simulink model "foc"  (R2021b)
settings: Solver=FixedStepAuto  StartTime=0.0  StopTime=20  FixedStep=Ts  MaxStep=1e-4  RelTol=1e-3
values from neighbouring files (symbols this model uses):
  currt_width = 200.0    [motor_parameters.sldd]
  Flux = 0.00103001    [motor_parameters.sldd]
  Gamma = 800000.0    [motor_parameters.sldd]
  Ibus = 5.0    [motor_parameters.sldd]
  Ls = 2.235E-5    [motor_parameters.sldd]
  Pn = 7.0    [motor_parameters.sldd]
  Rs = 0.112    [motor_parameters.sldd]
  Ts = 0.0001    [motor_parameters.sldd]
  Ubus = 12.0    [motor_parameters.sldd]
undefined symbols (not defined in the file or in its folder): DiscIntNeverNeededParam, magnitude, sigbuilder_block, spd_ki, spd_kp
libraries: slpidlib x4, mcbplantlib x1, simulink x1, autolibpmsmexterior x1
settings Model: DataDictionary=motor_parameters.sldd  Creator=chenpeng  LastModifiedBy=chenpeng
settings SolverCC: AutoInsertRateTranBlk=on
settings OptimizationCC: DefaultParameterBehavior=Inlined  UseDivisionForNetSlopeComputation=on  GainParamInheritBuiltInType=on  UseFloatMulNetSlope=on  InlineInvariantSignals=on  PassReuseOutputArgsAs=Individual arguments  ZeroExternalMemoryAtStartup=off  ZeroInternalMemoryAtStartup=off  NoFixptDivByZeroProtection=on  EfficientFloat2IntCast=on  LifeSpan=1  OptimizeBlockOrder=speed  DifferentSizesBufferReuse=on  EfficientTunableParamExpr=on
settings DebuggingCC: ParameterTunabilityLossMsg=error
settings HardwareCC: ProdBitPerPointer=32  ProdBitPerSizeT=32  ProdBitPerPtrDiffT=32  ProdLargestAtomicInteger=Long  ProdLargestAtomicFloat=Double  ProdWordSize=32  ProdLongLongMode=on  ProdHWDeviceType=ARM Compatible->ARM Cortex-M
settings SFSimCC: MATLABDynamicMemAlloc=off
settings RTWCC: Description=Embedded Coder  SystemTargetFile=ert.tlc  GenCodeOnly=on  TemplateMakefile=ert_default_tmf  Toolchain=GNU Tools for ARM Embedded Processors
settings CodeAppCC: ForceParamTrailComments=on  IgnoreCustomStorageClasses=off  OperatorAnnotations=on  SimulinkDataObjDesc=on  SFDataObjDesc=on  CustomSymbolStrGlobalVar=rt$N$M  CustomSymbolStrType=$N$M  CustomSymbolStrFcn=$N$M$F  CustomSymbolStrMacro=$N$M  InsertBlockDesc=on
settings ERTTargetCC: TargetLangStandard=C99 (ISO)  GenerateSampleERTMain=on  IncludeMdlTerminateFcn=off  CombineSignalStateStructs=on  SupportComplex=off  SupportNonInlinedSFcns=on  InlinedParameterPlacement=NonHierarchical  ERTCustomFileTemplate=example_file_process.tlc  ERTFilePackagingFormat=CompactWithDataFile

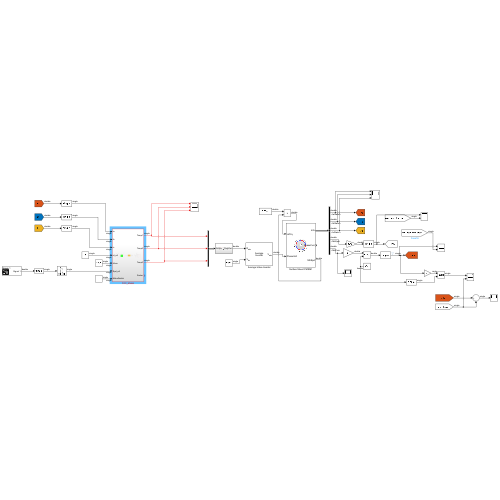
[thumbnail: Simulink's stored preview of the top-level diagram]
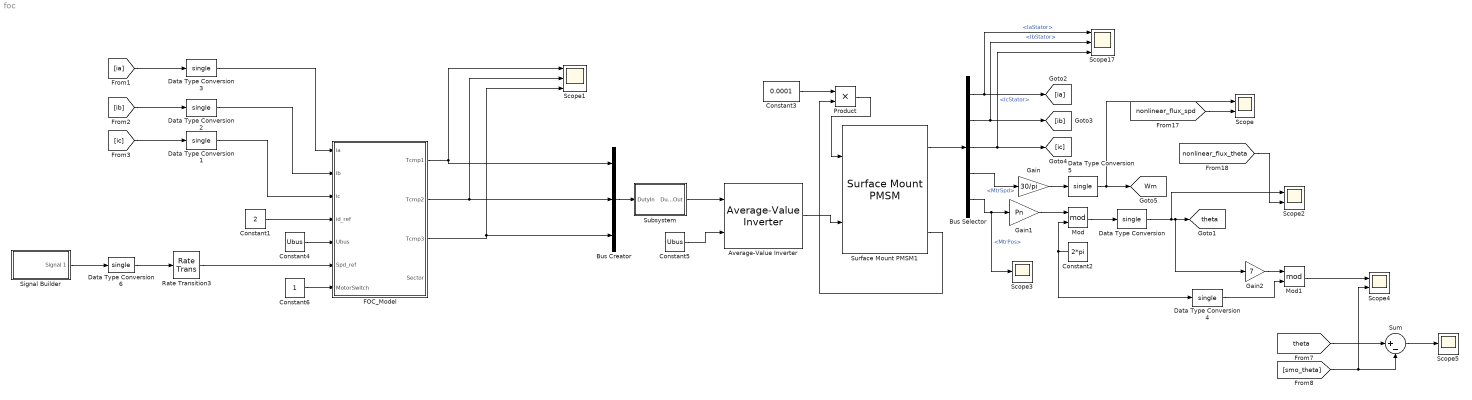
== system foc ==
  Average-Value Inverter : mcbplantlib/Average-Value Inverter
  Bus Creator : BusCreator  Inputs=3
  Bus Selector : BusSelector  OutputSignals=IaStator,IbStator,IcStator,MtrSpd,MtrPos
  Constant1 : Constant  Value=2  OutDataTypeStr=single  SampleTime=-1
  Constant2 : Constant  Value=2*pi
  Constant3 : Constant  Value=0.0001  OutDataTypeStr=double
  Constant4 : Constant  Value=Ubus  OutDataTypeStr=single
  Constant5 : Constant  Value=Ubus  OutDataTypeStr=single
  Constant6 : Constant  OutDataTypeStr=single  SampleTime=-1
  Data Type Conversion{,1..6} (7 alike) : DataTypeConversion  OutDataTypeStr=single
  FOC_Model : Subsystem
  Gain : Gain  Gain=30/pi
  Gain1 : Gain  Gain=Pn
  Gain2 : Gain  Gain=7
  Mod : Math  Operator=mod  SaturateOnIntegerOverflow=on
  Mod1 : Math  Operator=mod  SaturateOnIntegerOverflow=on
  Product : Product
  Rate Transition3 : RateTransition
  Scope : Scope  NumInputPorts=2
  Scope1 : Scope  NumInputPorts=3
  Scope17 : Scope  NumInputPorts=3
  Scope2 : Scope  NumInputPorts=2
  Scope3 : Scope
  Scope4 : Scope  NumInputPorts=2
  Scope5 : Scope
  Signal Builder : Subsystem  Tag=STV Subsys  LoadFcn=sigbuilder_block('load');  StartFcn=sigbuilder_block('start');  StopFcn=sigbuilder_block('stop');  ClipboardFcn=sigbuilder_block('clipboard');  mask(Sigbuilder block){tuvar=[0:10]}
      mask help: Simulink:masks:SigbuilderBlock_MD
      mask init:
      | if ~strcmp(get_param(bdroot(gcbh),'SimulationStatus'),'stopped') tuvar = sigbuilder_block('maskInit'); end
      settings: CopyFcn=sigbuilder_block('copy');  DeleteFcn=sigbuilder_block('delete');  ModelCloseFcn=sigbuilder_block('modelClose');  PreSaveFcn=sigbuilder_block('preSave');  PauseFcn=sigbuilder_block('pause');  ContinueFcn=sigbuilder_block('continue');  NameChangeFcn=sigbuilder_block('namechange');  OpenFcn=sigbuilder_block('open',[437.6 199.2 550.4 400 ]);  CloseFcn=sigbuilder_block('close');
      mask Display: plot(0, 0, 100, 100,[2, 2, 32, 32, 2], [68, 8, 8, 68, 68],[32, 2], [38, 38], [32, 19, 2],[53, 60, 44], [32, 17, 17, 2],[16, 16, 31, 31]);txt = getActiveGroup(gcbh);text(2, 100, txt,'verticalAlignment', 'top');
  Subsystem : Subsystem
  Sum : Sum  Inputs=|+-
  Surface Mount PMSM1 : autolibpmsmexterior/Surface Mount PMSM  port_config=Torque  sim_type=Discrete  Ts=Ts  FilePath=E:\Sandbox\Bauto\Work\surfacepmsm_motordata.m  P=Pn  Rs=Rs  Ldq_=Ls  KConstText=Permanent flux linkage constant (lambda_pm):  lambda_pm=Flux  Ke=159.9771  Kt=1.323  mechanical=[0.0027, 4.924e-4, 0]  idq0=[0 0]  theta_init=0  omega_init=0  KConst=Flux  lambda_pm_calc=Flux  RefBlkName='autolibpmsmexterior/Surface Mount PMSM'  aMode=1  Ldq="[0.0003752   0.0003752]"
      settings: SourceProductBaseCode=PW,DR,MT,UV,VE
  tag scope: Wm=global, theta=global
  wires:
  Data Type Conversion/1 -> Scope2/1, Gain2/1, [theta]
  Bus Selector/3 -> Scope17/3, [ic]  "<IcStator>"
  Mod/1 -> Data Type Conversion/1
  Gain/1 -> Data Type Conversion5/1
  Constant3/1 -> Product/1
  Gain1/1 -> Mod/1
  Data Type Conversion5/1 -> Scope/1, [Wm]
  Bus Creator/1 -> Subsystem/1(DutyIn)
  Bus Selector/5 -> Scope3/1, Gain1/1  "<MtrPos>"
  Bus Selector/1 -> [ia], Scope17/1  "<IaStator>"
  Subsystem/1(DutyOut) -> Average-Value Inverter/1
  Bus Selector/2 -> Scope17/2, [ib]  "<IbStator>"
  Bus Selector/4 -> Gain/1  "<MtrSpd>"
  Constant2/1 -> Data Type Conversion4/1, Mod/2
  Constant5/1 -> Average-Value Inverter/2
  [ia] -> Data Type Conversion3/1
  [ib] -> Data Type Conversion2/1
  [ic] -> Data Type Conversion1/1
  Average-Value Inverter/1 -> Surface Mount PMSM1/2
  Surface Mount PMSM1/3 -> Product/2
  Surface Mount PMSM1/1 -> Bus Selector/1
  Gain2/1 -> Mod1/1
  Mod1/1 -> Scope4/1
  Data Type Conversion4/1 -> Mod1/2
  Product/1 -> Surface Mount PMSM1/1
  Data Type Conversion3/1 -> FOC_Model/1(ia)
  Data Type Conversion2/1 -> FOC_Model/2(ib)
  Data Type Conversion1/1 -> FOC_Model/3(ic)
  Constant4/1 -> FOC_Model/5(Ubus)
  FOC_Model/1(Tcmp1) -> Bus Creator/1, Scope1/1
  FOC_Model/2(Tcmp2) -> Scope1/2, Bus Creator/2
  FOC_Model/3(Tcmp3) -> Scope1/3, Bus Creator/3
  Constant6/1 -> FOC_Model/7(MotorSwitch)
  Constant1/1 -> FOC_Model/4(id_ref)
  [smo_theta] -> Scope4/2, Sum/2
  Sum/1 -> Scope5/1
  Data Type Conversion6/1 -> Rate Transition3/1
  Signal Builder/1(Signal 1) -> Data Type Conversion6/1
  [theta] -> Sum/1
  [nonlinear_flux_spd] -> Scope/2
  [nonlinear_flux_theta] -> Scope2/2
  Rate Transition3/1 -> FOC_Model/6(Spd_ref)

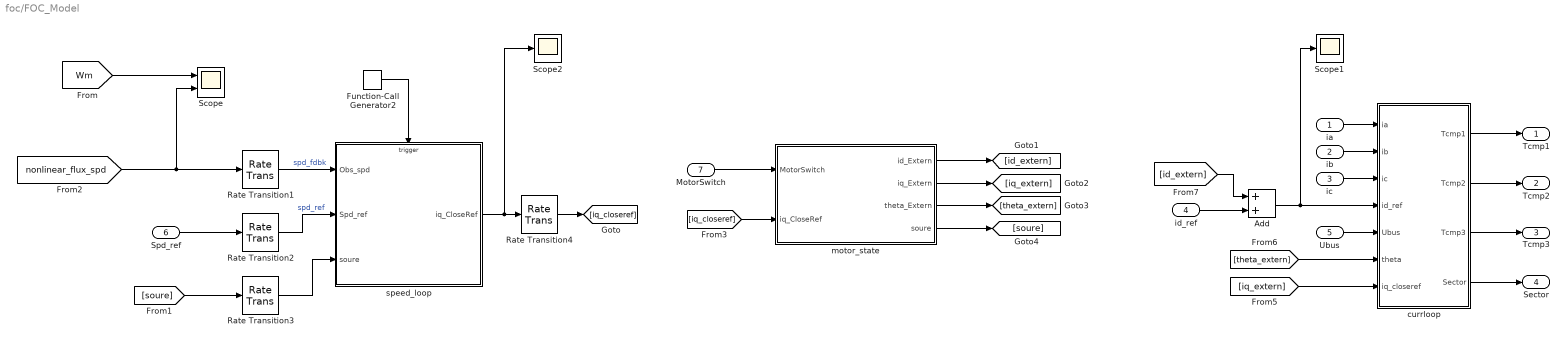
== system foc/FOC_Model ==
  ia : Inport  OutDataTypeStr=single
  ib : Inport  Port=2  OutDataTypeStr=single
  ic : Inport  Port=3  OutDataTypeStr=single
  id_ref : Inport  Port=4  OutDataTypeStr=single
  Ubus : Inport  Port=5  OutDataTypeStr=single
  Spd_ref : Inport  Port=6  OutDataTypeStr=single
  MotorSwitch : Inport  Port=7  OutDataTypeStr=single
  Add : Sum
  Function-Call Generator2 : simulink/Ports & Subsystems/Function-Call Generator  sample_time=1e-3  numberOfIterations=1  DisallowWideOutput=off
  Rate Transition{1..4} (4 alike) : RateTransition
  Scope : Scope  NumInputPorts=2
  Scope1 : Scope
  Scope2 : Scope
  currloop : Subsystem
  motor_state : Subsystem
  speed_loop : Subsystem  TreatAsAtomicUnit=on  SystemSampleTime=1e-4
      settings: RTWSystemCode=Nonreusable function  RTWFcnNameOpts=Use subsystem name
  Tcmp1 : Outport  OutDataTypeStr=single
  Tcmp2 : Outport  Port=2  OutDataTypeStr=single
  Tcmp3 : Outport  Port=3  OutDataTypeStr=single
  Sector : Outport  Port=4  OutDataTypeStr=single
  wires:
  Rate Transition1/1 -> speed_loop/1(Obs_spd)  "spd_fdbk"
  ia/1 -> currloop/1(ia)
  ib/1 -> currloop/2(ib)
  Ubus/1 -> currloop/5(Ubus)
  currloop/4(Sector) -> Sector/1
  currloop/2(Tcmp2) -> Tcmp2/1
  Rate Transition2/1 -> speed_loop/2(Spd_ref)  "spd_ref"
  speed_loop/1(iq_CloseRef) -> Scope2/1, Rate Transition4/1
  ic/1 -> currloop/3(ic)
  currloop/1(Tcmp1) -> Tcmp1/1
  currloop/3(Tcmp3) -> Tcmp3/1
  Spd_ref/1 -> Rate Transition2/1
  [Wm] -> Scope/1
  [nonlinear_flux_spd] -> Scope/2, Rate Transition1/1
  Rate Transition3/1 -> speed_loop/3(soure)
  [soure] -> Rate Transition3/1
  MotorSwitch/1 -> motor_state/1(MotorSwitch)
  Rate Transition4/1 -> [iq_closeref]
  [iq_closeref] -> motor_state/2(iq_CloseRef)
  motor_state/1(id_Extern) -> [id_extern]
  id_ref/1 -> Add/2
  [id_extern] -> Add/1
  Add/1 -> Scope1/1, currloop/4(id_ref)
  motor_state/2(iq_Extern) -> [iq_extern]
  motor_state/4(soure) -> [soure]
  [iq_extern] -> currloop/7(iq_closeref)
  [theta_extern] -> currloop/6(theta)
  motor_state/3(theta_Extern) -> [theta_extern]
  Function-Call Generator2/1 -> speed_loop/Trigger

== system foc/Signal Builder ==
  Demux : Demux  Tag=STV Demux  Outputs=1
      settings: DisplayOption=none
  FromWs : FromWorkspace  Tag=STV FromWs  VariableName=tuvar
      SigBuilderData=|
      | common.afterFinalStr = 'Extrapolate'
      | common.sampleTime = 0
      | dataSet.timeRange = [0 10]
      | dataSet.name = 'Group 1'
      | sbobj.Groups.Name = 'Group 1'
      | sbobj.Groups.Signals.Name = 'Signal 1'
      | sbobj.Groups.Signals.XData = [0 4 4 7 7 10]
      | sbobj.Groups.Signals.YData = [200 200 598 602 800 802]
  Signal 1 : Outport  Tag=STV Outport
  wires:
  Demux/1 -> Signal 1/1
  FromWs/1 -> Demux/1

== system foc/Subsystem ==
  DutyIn : Inport
  Constant : Constant  Value=0.5  OutDataTypeStr=double  SampleTime=-1
  Gain : Gain  Gain=1/8000  ParamDataTypeStr=single
  Gain1 : Gain  Gain=-1
  Sum : Sum  Inputs=|+-
  Sum1 : Sum  Inputs=|++
  DutyOut : Outport
  wires:
  Sum/1 -> Gain1/1
  Constant/1 -> Sum1/2, Sum/2
  DutyIn/1 -> Gain/1
  Gain1/1 -> Sum1/1
  Sum1/1 -> DutyOut/1
  Gain/1 -> Sum/1

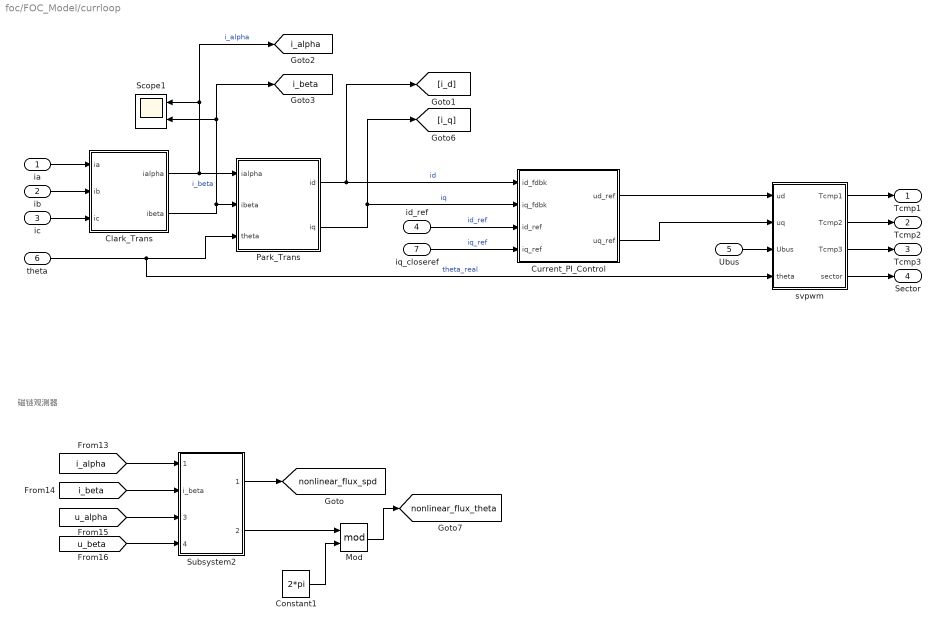
== system foc/FOC_Model/currloop ==
  note: 磁链观测器
  ia : Inport  OutDataTypeStr=single  SampleTime=0.0001
  ib : Inport  Port=2  OutDataTypeStr=single  SampleTime=0.0001
  ic : Inport  Port=3  OutDataTypeStr=single  SampleTime=0.0001
  id_ref : Inport  Port=4  OutDataTypeStr=single  SampleTime=0.0001
  Ubus : Inport  Port=5  SampleTime=0.0001
  theta : Inport  Port=6  OutDataTypeStr=single  SampleTime=0.0001
  iq_closeref : Inport  Port=7  OutDataTypeStr=single  SampleTime=0.0001
  Clark_Trans : Subsystem  TreatAsAtomicUnit=on
  Constant1 : Constant  Value=2*pi  OutDataTypeStr=single
  Current_PI_Control : Subsystem
  Mod : Math  Operator=mod  SaturateOnIntegerOverflow=on
  Park_Trans : Subsystem  TreatAsAtomicUnit=on
  Scope1 : Scope  NumInputPorts=2
  Subsystem2 : Subsystem
  svpwm : Subsystem
  Tcmp1 : Outport
  Tcmp2 : Outport  Port=2
  Tcmp3 : Outport  Port=3
  Sector : Outport  Port=4
  tag scope: i_alpha=global, i_beta=global, nonlinear_flux_spd=global, nonlinear_flux_theta=global
  wires:
  Park_Trans/2(iq) -> Current_PI_Control/2(iq_fdbk), [i_q]  "iq"
  ia/1 -> Clark_Trans/1(ia)
  ic/1 -> Clark_Trans/3(ic)
  Park_Trans/1(id) -> [i_d], Current_PI_Control/1(id_fdbk)  "id"
  ib/1 -> Clark_Trans/2(ib)
  svpwm/1(Tcmp1) -> Tcmp1/1
  svpwm/2(Tcmp2) -> Tcmp2/1
  svpwm/3(Tcmp3) -> Tcmp3/1
  svpwm/4(sector) -> Sector/1
  Ubus/1 -> svpwm/3(Ubus)
  id_ref/1 -> Current_PI_Control/3(id_ref)  "id_ref"
  Clark_Trans/2(ibeta) -> [i_beta], Scope1/2, Park_Trans/2(ibeta)  "i_beta"
  Clark_Trans/1(ialpha) -> [i_alpha], Scope1/1, Park_Trans/1(ialpha)  "i_alpha"
  theta/1 -> svpwm/4(theta), Park_Trans/3(theta)  "theta_real"
  iq_closeref/1 -> Current_PI_Control/4(iq_ref)  "iq_ref"
  Current_PI_Control/2(uq_ref) -> svpwm/2(uq)
  Current_PI_Control/1(ud_ref) -> svpwm/1(ud)
  Subsystem2/1(Output) -> [nonlinear_flux_spd]
  [i_alpha] -> Subsystem2/1(i_alpha)
  [i_beta] -> Subsystem2/2(i_beta)
  [u_alpha] -> Subsystem2/3(u_alpha)
  [u_beta] -> Subsystem2/4(u_beta)
  Subsystem2/2(Output1) -> Mod/1
  Constant1/1 -> Mod/2
  Mod/1 -> [nonlinear_flux_theta]

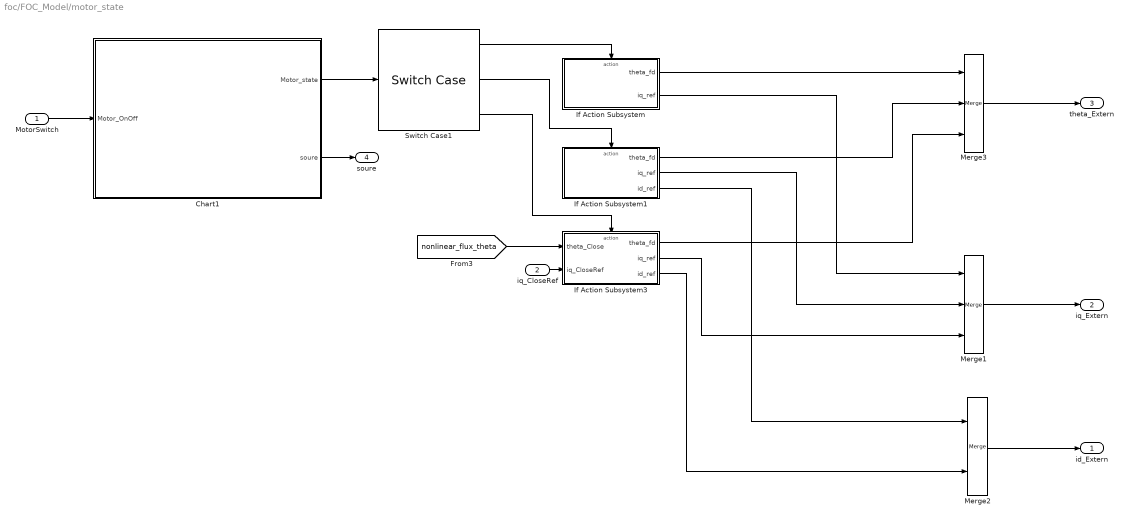
== system foc/FOC_Model/motor_state ==
  MotorSwitch : Inport  OutDataTypeStr=single
  iq_CloseRef : Inport  Port=2
  Chart1 : Stateflow chart  TreatAsAtomicUnit=on
  If Action Subsystem : Subsystem  TreatAsAtomicUnit=on
  If Action Subsystem1 : Subsystem  TreatAsAtomicUnit=on
  If Action Subsystem3 : Subsystem  TreatAsAtomicUnit=on
  Merge1 : Merge  Inputs=3
  Merge2 : Merge
  Merge3 : Merge  Inputs=3
  Switch Case1 : SwitchCase  CaseConditions={1,2,3}  ShowDefaultCase=off
  id_Extern : Outport
  iq_Extern : Outport  Port=2
  theta_Extern : Outport  Port=3
  soure : Outport  Port=4  OutDataTypeStr=single
  wires:
  Switch Case1/3 -> If Action Subsystem3/Action
  If Action Subsystem/1(theta_fd) -> Merge3/1
  If Action Subsystem1/2(iq_ref) -> Merge1/2
  If Action Subsystem3/3(id_ref) -> Merge2/2
  Switch Case1/2 -> If Action Subsystem1/Action
  If Action Subsystem3/2(iq_ref) -> Merge1/3
  If Action Subsystem1/1(theta_fd) -> Merge3/2
  Chart1/2(soure) -> soure/1
  MotorSwitch/1 -> Chart1/1(Motor_OnOff)
  Chart1/1(Motor_state) -> Switch Case1/1
  If Action Subsystem1/3(id_ref) -> Merge2/1
  If Action Subsystem3/1(theta_fd) -> Merge3/3
  Switch Case1/1 -> If Action Subsystem/Action
  If Action Subsystem/2(iq_ref) -> Merge1/1
  iq_CloseRef/1 -> If Action Subsystem3/2(iq_CloseRef)
  [nonlinear_flux_theta] -> If Action Subsystem3/1(theta_Close)
  Merge3/1 -> theta_Extern/1
  Merge1/1 -> iq_Extern/1
  Merge2/1 -> id_Extern/1

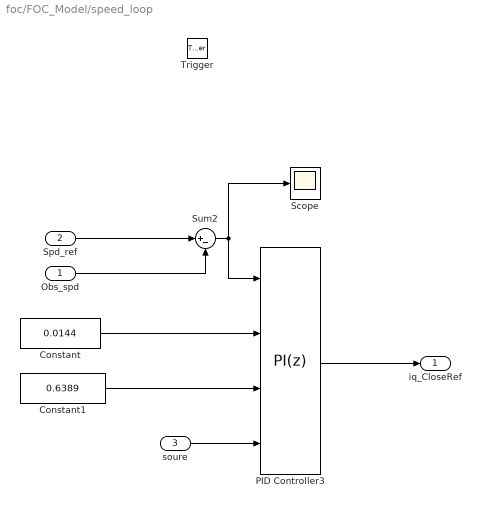
== system foc/FOC_Model/speed_loop ==
  Obs_spd : Inport  OutDataTypeStr=single  PortDimensions=1
  Spd_ref : Inport  Port=2  OutDataTypeStr=single  PortDimensions=1
  soure : Inport  Port=3  OutDataTypeStr=single  PortDimensions=1
  Trigger : TriggerPort  TriggerType=function-call  VariantControl=(inherit)  PortDimensions=1
  Constant : Constant  Value=0.0144  OutDataTypeStr=single  SampleTime=-1
  Constant1 : Constant  Value=0.6389  OutDataTypeStr=single  SampleTime=-1
  PID Controller3 : slpidlib/PID Controller  Controller=PI  Form=Parallel  TimeDomain=Discrete-time  UseExternalTs=off  SampleTime=-1  IntegratorMethod=Forward Euler  FilterMethod=Forward Euler  ControllerParametersSource=external  P=spd_kp  I=spd_ki  D=0  UseFilter=on  N=100  TunerSelectOption=Transfer Function Based (PID Tuner App)  InitialConditionSource=internal  InitialConditionForIntegrator=0  InitialConditionForFilter=0  DifferentiatorICPrevScaledInput=0  ExternalReset=rising  TrackingMode=off  Kt=1  LimitOutput=on  SatLimitsSource=internal  UpperSaturationLimit=Ibus  LowerSaturationLimit=-Ibus  LinearizeAsGain=on  AntiWindupMode=clamping  Kb=0.013  PGainOutDataTypeStr=single  PProdOutDataTypeStr=single  POutMin=[]  POutMax=[]  IGainOutDataTypeStr=single  IProdOutDataTypeStr=single  IOutMin=[]  IOutMax=[]  DOutMin=[]  DOutMax=[]  NOutMin=[]  NOutMax=[]  SumOutDataTypeStr=single  SumOutMin=[]  SumOutMax=[]  SaturationOutDataTypeStr=single  SaturationOutMin=[]  SaturationOutMax=[]  PParamMin=[]  PParamMax=[]  IParamMin=[]  IParamMax=[]  DParamMin=[]  DParamMax=[]  NParamMin=[]  NParamMax=[]  KbParamMin=[]  KbParamMax=[]  KtParamMin=[]  KtParamMax=[]  KbOutMin=[]  KbOutMax=[]  KtOutMin=[]  KtOutMax=[]  IntegratorOutMin=[]  IntegratorOutMax=[]  FilterOutMin=[]  FilterOutMax=[]  SumI1OutMin=[]  SumI1OutMax=[]  SumI2OutMin=[]  SumI2OutMax=[]  SumI3OutMin=[]  SumI3OutMax=[]  SumI4OutMin=[]  SumI4OutMax=[]  SumDOutMin=[]  SumDOutMax=[]  DifferentiatorOutMin=[]  DifferentiatorOutMax=[]  FilterDiffOutCoefMin=[]  FilterDiffOutCoefMax=[]  ReciprocalOutMin=[]  ReciprocalOutMax=[]  SumDenOutMin=[]  SumDenOutMax=[]  SumNumOutMin=[]  SumNumOutMax=[]  DivideOutMin=[]  DivideOutMax=[]  UdiffTsProdOutMin=[]  UdiffTsProdOutMax=[]  NTsProdOutMin=[]  NTsProdOutMax=[]  UintegralTsProdOutMin=[]  UintegralTsProdOutMax=[]  UngainTsProdOutMin=[]  UngainTsProdOutMax=[]  IntegratorContinuousStateAttributes=''  IntegratorStateMustResolveToSignalObject=off  IntegratorRTWStateStorageClass=Auto  FilterContinuousStateAttributes=''  FilterStateMustResolveToSignalObject=off  FilterRTWStateStorageClass=Auto  ParallelPVariant=ExternalParameters  IdealPVariant=Disabled  IVariant=ExternalParameters  DVariant=Disabled  IntegratorVariant=Discrete  SatVariant=Enabled  AWVariant=DiscClampingParallel  PCopyVariant=Disabled  TRVariant=Disabled  FdbkBlocksVariant=Forward  IdealPFdbkVariant=Disabled  SatFdbkVariant=Disabled  DerivativeFilterVariant=Disabled  NVariant=Disabled  NCopyVariant=Disabled_SignalSpec  FilterICVariant=Disabled  IntegratorICVariant=InternalICs  ExternalResetVariant=ExternalReset  TRSumVariant=Passthrough  SumFdbkVariant=Disabled  SumVariant=Sum_PI  TsampFilterVariant=InternalTs  TsampNgainVariant=Passthrough  TsampIntegralVariant=Passthrough  ExternalSaturationOutDataTypeStr=single
  Scope : Scope
  Sum2 : Sum  Inputs=|+-  AccumDataTypeStr=single  OutDataTypeStr=single
  iq_CloseRef : Outport
  wires:
  Obs_spd/1 -> Sum2/2
  Spd_ref/1 -> Sum2/1
  Sum2/1 -> Scope/1, PID Controller3/1
  PID Controller3/1 -> iq_CloseRef/1
  Constant/1 -> PID Controller3/2
  Constant1/1 -> PID Controller3/3
  soure/1 -> PID Controller3/4

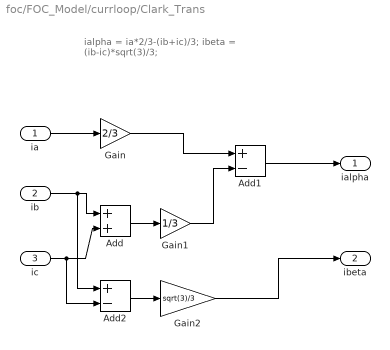
== system foc/FOC_Model/currloop/Clark_Trans ==
  note: ialpha = ia*2/3-(ib+ic)/3;
      | ibeta = (ib-ic)*sqrt(3)/3;
  ia : Inport  OutDataTypeStr=single
  ib : Inport  Port=2  OutDataTypeStr=single
  ic : Inport  Port=3  OutDataTypeStr=single
  Add : Sum  AccumDataTypeStr=single  OutDataTypeStr=single
  Add1 : Sum  Inputs=+-  AccumDataTypeStr=single  OutDataTypeStr=single
  Add2 : Sum  Inputs=+-  AccumDataTypeStr=single  OutDataTypeStr=single
  Gain : Gain  Gain=2/3  ParamDataTypeStr=single
  Gain1 : Gain  Gain=1/3  ParamDataTypeStr=single
  Gain2 : Gain  Gain=sqrt(3)/3  ParamDataTypeStr=single
  ialpha : Outport  OutDataTypeStr=single
  ibeta : Outport  Port=2  OutDataTypeStr=single
  wires:
  ia/1 -> Gain/1
  ib/1 -> Add2/1, Add/1
  ic/1 -> Add2/2, Add/2
  Add/1 -> Gain1/1
  Gain/1 -> Add1/1
  Gain1/1 -> Add1/2
  Add1/1 -> ialpha/1
  Add2/1 -> Gain2/1
  Gain2/1 -> ibeta/1

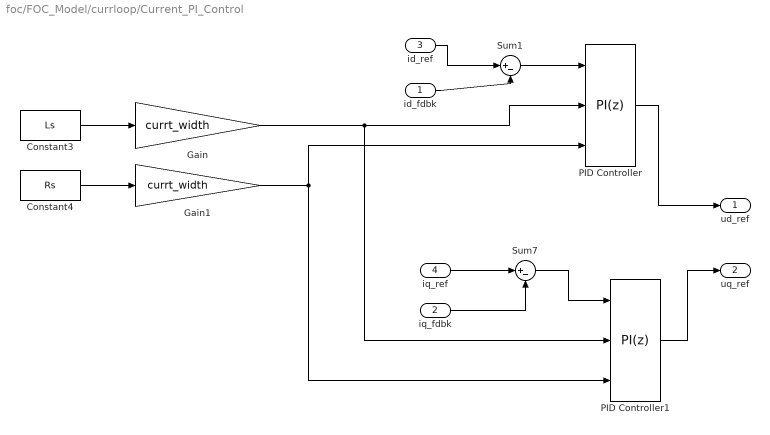
== system foc/FOC_Model/currloop/Current_PI_Control ==
  id_fdbk : Inport  OutDataTypeStr=single
  iq_fdbk : Inport  Port=2  OutDataTypeStr=single
  id_ref : Inport  Port=3  OutDataTypeStr=single
  iq_ref : Inport  Port=4  OutDataTypeStr=single
  Constant3 : Constant  Value=Ls  OutDataTypeStr=single  SampleTime=-1
  Constant4 : Constant  Value=Rs  OutDataTypeStr=single  SampleTime=-1
  Gain : Gain  Gain=currt_width  OutDataTypeStr=single
  Gain1 : Gain  Gain=currt_width  OutDataTypeStr=single
  PID Controller : slpidlib/PID Controller  Controller=PI  Form=Parallel  TimeDomain=Discrete-time  UseExternalTs=off  SampleTime=-1  IntegratorMethod=Forward Euler  FilterMethod=Forward Euler  ControllerParametersSource=external  P=1  I=1  D=0  UseFilter=on  N=100  TunerSelectOption=Transfer Function Based (PID Tuner App)  InitialConditionSource=internal  InitialConditionForIntegrator=0  InitialConditionForFilter=0  DifferentiatorICPrevScaledInput=0  ExternalReset=none  TrackingMode=off  Kt=1  LimitOutput=on  SatLimitsSource=internal  UpperSaturationLimit=Ubus*0.9/sqrt(3)  LowerSaturationLimit=-Ubus*0.9/sqrt(3)  LinearizeAsGain=on  AntiWindupMode=none  Kb=1  POutMin=[]  POutMax=[]  IOutMin=[]  IOutMax=[]  DOutMin=[]  DOutMax=[]  NOutMin=[]  NOutMax=[]  SumOutMin=[]  SumOutMax=[]  SaturationOutMin=[]  SaturationOutMax=[]  PParamMin=[]  PParamMax=[]  IParamMin=[]  IParamMax=[]  DParamMin=[]  DParamMax=[]  NParamMin=[]  NParamMax=[]  KbParamMin=[]  KbParamMax=[]  KtParamMin=[]  KtParamMax=[]  KbOutMin=[]  KbOutMax=[]  KtOutMin=[]  KtOutMax=[]  IntegratorOutMin=[]  IntegratorOutMax=[]  FilterOutMin=[]  FilterOutMax=[]  SumI1OutMin=[]  SumI1OutMax=[]  SumI2OutMin=[]  SumI2OutMax=[]  SumI3OutMin=[]  SumI3OutMax=[]  SumI4OutMin=[]  SumI4OutMax=[]  SumDOutMin=[]  SumDOutMax=[]  DifferentiatorOutMin=[]  DifferentiatorOutMax=[]  FilterDiffOutCoefMin=[]  FilterDiffOutCoefMax=[]  ReciprocalOutMin=[]  ReciprocalOutMax=[]  SumDenOutMin=[]  SumDenOutMax=[]  SumNumOutMin=[]  SumNumOutMax=[]  DivideOutMin=[]  DivideOutMax=[]  UdiffTsProdOutMin=[]  UdiffTsProdOutMax=[]  NTsProdOutMin=[]  NTsProdOutMax=[]  UintegralTsProdOutMin=[]  UintegralTsProdOutMax=[]  UngainTsProdOutMin=[]  UngainTsProdOutMax=[]  IntegratorContinuousStateAttributes=''  IntegratorStateMustResolveToSignalObject=off  IntegratorRTWStateStorageClass=Auto  FilterContinuousStateAttributes=''  FilterStateMustResolveToSignalObject=off  FilterRTWStateStorageClass=Auto  ParallelPVariant=ExternalParameters  IdealPVariant=Disabled  IVariant=ExternalParameters  DVariant=Disabled  IntegratorVariant=Discrete  SatVariant=Enabled  AWVariant=Passthrough  PCopyVariant=Disabled  TRVariant=Disabled  FdbkBlocksVariant=Forward  IdealPFdbkVariant=Disabled  SatFdbkVariant=Disabled  DerivativeFilterVariant=Disabled  NVariant=Disabled  NCopyVariant=Disabled_SignalSpec  FilterICVariant=Disabled  IntegratorICVariant=InternalICs  ExternalResetVariant=Disabled  TRSumVariant=Passthrough  SumFdbkVariant=Disabled  SumVariant=Sum_PI  TsampFilterVariant=InternalTs  TsampNgainVariant=Passthrough  TsampIntegralVariant=Passthrough  ExternalSaturationOutDataTypeStr=Inherit: Same as second input
  PID Controller1 : slpidlib/PID Controller  Controller=PI  Form=Parallel  TimeDomain=Discrete-time  UseExternalTs=off  SampleTime=-1  IntegratorMethod=Forward Euler  FilterMethod=Forward Euler  ControllerParametersSource=external  P=1  I=1  D=0  UseFilter=on  N=100  TunerSelectOption=Transfer Function Based (PID Tuner App)  InitialConditionSource=internal  InitialConditionForIntegrator=0  InitialConditionForFilter=0  DifferentiatorICPrevScaledInput=0  ExternalReset=none  TrackingMode=off  Kt=1  LimitOutput=on  SatLimitsSource=internal  UpperSaturationLimit=Ubus*0.9/sqrt(3)  LowerSaturationLimit=-Ubus*0.9/sqrt(3)  LinearizeAsGain=on  AntiWindupMode=none  Kb=1  POutMin=[]  POutMax=[]  IOutMin=[]  IOutMax=[]  DOutMin=[]  DOutMax=[]  NOutMin=[]  NOutMax=[]  SumOutMin=[]  SumOutMax=[]  SaturationOutMin=[]  SaturationOutMax=[]  PParamMin=[]  PParamMax=[]  IParamMin=[]  IParamMax=[]  DParamMin=[]  DParamMax=[]  NParamMin=[]  NParamMax=[]  KbParamMin=[]  KbParamMax=[]  KtParamMin=[]  KtParamMax=[]  KbOutMin=[]  KbOutMax=[]  KtOutMin=[]  KtOutMax=[]  IntegratorOutMin=[]  IntegratorOutMax=[]  FilterOutMin=[]  FilterOutMax=[]  SumI1OutMin=[]  SumI1OutMax=[]  SumI2OutMin=[]  SumI2OutMax=[]  SumI3OutMin=[]  SumI3OutMax=[]  SumI4OutMin=[]  SumI4OutMax=[]  SumDOutMin=[]  SumDOutMax=[]  DifferentiatorOutMin=[]  DifferentiatorOutMax=[]  FilterDiffOutCoefMin=[]  FilterDiffOutCoefMax=[]  ReciprocalOutMin=[]  ReciprocalOutMax=[]  SumDenOutMin=[]  SumDenOutMax=[]  SumNumOutMin=[]  SumNumOutMax=[]  DivideOutMin=[]  DivideOutMax=[]  UdiffTsProdOutMin=[]  UdiffTsProdOutMax=[]  NTsProdOutMin=[]  NTsProdOutMax=[]  UintegralTsProdOutMin=[]  UintegralTsProdOutMax=[]  UngainTsProdOutMin=[]  UngainTsProdOutMax=[]  IntegratorContinuousStateAttributes=''  IntegratorStateMustResolveToSignalObject=off  IntegratorRTWStateStorageClass=Auto  FilterContinuousStateAttributes=''  FilterStateMustResolveToSignalObject=off  FilterRTWStateStorageClass=Auto  ParallelPVariant=ExternalParameters  IdealPVariant=Disabled  IVariant=ExternalParameters  DVariant=Disabled  IntegratorVariant=Discrete  SatVariant=Enabled  AWVariant=Passthrough  PCopyVariant=Disabled  TRVariant=Disabled  FdbkBlocksVariant=Forward  IdealPFdbkVariant=Disabled  SatFdbkVariant=Disabled  DerivativeFilterVariant=Disabled  NVariant=Disabled  NCopyVariant=Disabled_SignalSpec  FilterICVariant=Disabled  IntegratorICVariant=InternalICs  ExternalResetVariant=Disabled  TRSumVariant=Passthrough  SumFdbkVariant=Disabled  SumVariant=Sum_PI  TsampFilterVariant=InternalTs  TsampNgainVariant=Passthrough  TsampIntegralVariant=Passthrough  ExternalSaturationOutDataTypeStr=Inherit: Same as second input
  Sum1 : Sum  Inputs=|+-  AccumDataTypeStr=single  OutDataTypeStr=single
  Sum7 : Sum  Inputs=|+-  AccumDataTypeStr=single  OutDataTypeStr=single
  ud_ref : Outport  OutDataTypeStr=single
  uq_ref : Outport  Port=2  OutDataTypeStr=single
  wires:
  id_fdbk/1 -> Sum1/2
  id_ref/1 -> Sum1/1
  iq_fdbk/1 -> Sum7/2
  Sum1/1 -> PID Controller/1
  Sum7/1 -> PID Controller1/1
  PID Controller/1 -> ud_ref/1
  PID Controller1/1 -> uq_ref/1
  iq_ref/1 -> Sum7/1
  Constant4/1 -> Gain1/1
  Constant3/1 -> Gain/1
  Gain/1 -> PID Controller1/2, PID Controller/2
  Gain1/1 -> PID Controller1/3, PID Controller/3

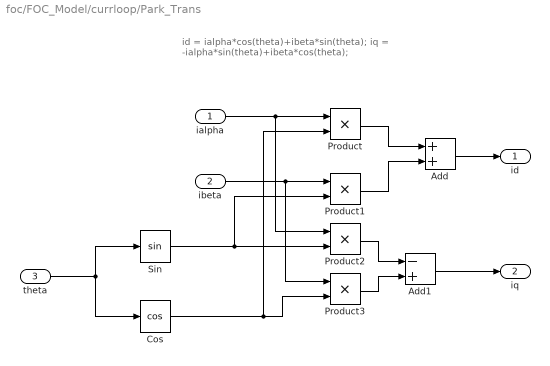
== system foc/FOC_Model/currloop/Park_Trans ==
  note: id = ialpha*cos(theta)+ibeta*sin(theta);
      | iq = -ialpha*sin(theta)+ibeta*cos(theta);
  ialpha : Inport  OutDataTypeStr=single
  ibeta : Inport  Port=2  OutDataTypeStr=single
  theta : Inport  Port=3  OutDataTypeStr=single
  Add : Sum  AccumDataTypeStr=single  OutDataTypeStr=single
  Add1 : Sum  Inputs=-+  AccumDataTypeStr=single  OutDataTypeStr=single
  Cos : Trigonometry  Operator=cos  ApproximationMethod=Lookup
  Product{,1..3} (4 alike) : Product  OutDataTypeStr=single
  Sin : Trigonometry  ApproximationMethod=Lookup
  id : Outport  OutDataTypeStr=single
  iq : Outport  Port=2  OutDataTypeStr=single
  wires:
  ialpha/1 -> Product2/1, Product/1
  ibeta/1 -> Product3/1, Product1/1
  Product/1 -> Add/1
  Product1/1 -> Add/2
  Add/1 -> id/1
  Product2/1 -> Add1/1
  Product3/1 -> Add1/2
  Add1/1 -> iq/1
  theta/1 -> Cos/1, Sin/1
  Sin/1 -> Product1/2, Product2/2
  Cos/1 -> Product/2, Product3/2

== system foc/FOC_Model/currloop/Subsystem2 ==
  i_alpha : Inport  OutDataTypeStr=single
  i_beta : Inport  Port=2  OutDataTypeStr=single
  u_alpha : Inport  Port=3  OutDataTypeStr=single
  u_beta : Inport  Port=4  OutDataTypeStr=single
  PLL : Subsystem
  noliner : Subsystem
  wm->Nr2 : Gain  Gain=30/(pi*Pn)  OutDataTypeStr=single
  Output : Outport  OutDataTypeStr=single
  Output1 : Outport  Port=2  OutDataTypeStr=single
  wires:
  noliner/1(cos) -> PLL/1(cos)
  PLL/2(theta) -> Output1/1  "flux_theta"
  PLL/1(Omega) -> wm->Nr2/1
  noliner/2(sin) -> PLL/2(sin)
  wm->Nr2/1 -> Output/1  "real"
  u_beta/1 -> noliner/4(u_beta)
  u_alpha/1 -> noliner/3(u_alpha)
  i_beta/1 -> noliner/2(i_beta)
  i_alpha/1 -> noliner/1(i_alpha)

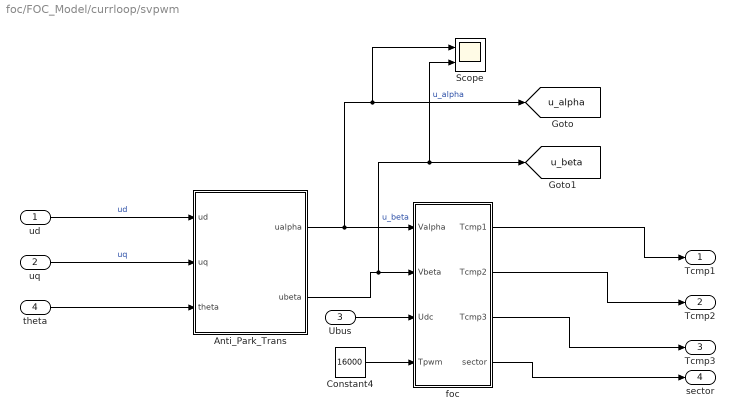
== system foc/FOC_Model/currloop/svpwm ==
  ud : Inport  OutDataTypeStr=single
  uq : Inport  Port=2
  Ubus : Inport  Port=3  SampleTime=0.0001
  theta : Inport  Port=4
  Anti_Park_Trans : Subsystem  TreatAsAtomicUnit=on
  Constant4 : Constant  Value=16000  OutDataTypeStr=single
  Scope : Scope  NumInputPorts=2
  foc : MATLAB Function  TreatAsAtomicUnit=on
  Tcmp1 : Outport
  Tcmp2 : Outport  Port=2
  Tcmp3 : Outport  Port=3
  sector : Outport  Port=4
  tag scope: u_alpha=global, u_beta=global
  wires:
  foc/1(Tcmp1) -> Tcmp1/1
  Constant4/1 -> foc/4(Tpwm)
  Ubus/1 -> foc/3(Udc)
  uq/1 -> Anti_Park_Trans/2(uq)  "uq"
  foc/4(sector) -> sector/1
  ud/1 -> Anti_Park_Trans/1(ud)  "ud"
  foc/3(Tcmp3) -> Tcmp3/1
  foc/2(Tcmp2) -> Tcmp2/1
  theta/1 -> Anti_Park_Trans/3(theta)
  Anti_Park_Trans/1(ualpha) -> Scope/1, [u_alpha], foc/1(Valpha)  "u_alpha"
  Anti_Park_Trans/2(ubeta) -> Scope/2, [u_beta], foc/2(Vbeta)  "u_beta"

== system foc/FOC_Model/motor_state/If Action Subsystem ==
  Action Port : ActionPort  ActionPortLabel=case [ 1 ]:
  Constant : Constant  Value=0  OutDataTypeStr=single  SampleTime=-1
  Constant1 : Constant  Value=0  OutDataTypeStr=single  SampleTime=-1
  theta_fd : Outport
  iq_ref : Outport  Port=2
  wires:
  Constant/1 -> theta_fd/1
  Constant1/1 -> iq_ref/1

== system foc/FOC_Model/motor_state/If Action Subsystem1 ==
  Action Port : ActionPort  ActionPortLabel=case [ 2 ]:
  Constant : Constant  Value=0  OutDataTypeStr=single  SampleTime=-1
  Constant1 : Constant  Value=0  OutDataTypeStr=single  SampleTime=-1
  Constant2 : Constant  Value=2  OutDataTypeStr=single  SampleTime=-1
  theta_fd : Outport
  iq_ref : Outport  Port=2
  id_ref : Outport  Port=3
  wires:
  Constant/1 -> theta_fd/1
  Constant1/1 -> iq_ref/1
  Constant2/1 -> id_ref/1

== system foc/FOC_Model/motor_state/If Action Subsystem3 ==
  theta_Close : Inport
  iq_CloseRef : Inport  Port=2
  Action Port : ActionPort  ActionPortLabel=case [ 3 ]:
  Constant2 : Constant  Value=0  OutDataTypeStr=single  SampleTime=-1
  theta_fd : Outport
  iq_ref : Outport  Port=2
  id_ref : Outport  Port=3
  wires:
  theta_Close/1 -> theta_fd/1
  iq_CloseRef/1 -> iq_ref/1
  Constant2/1 -> id_ref/1

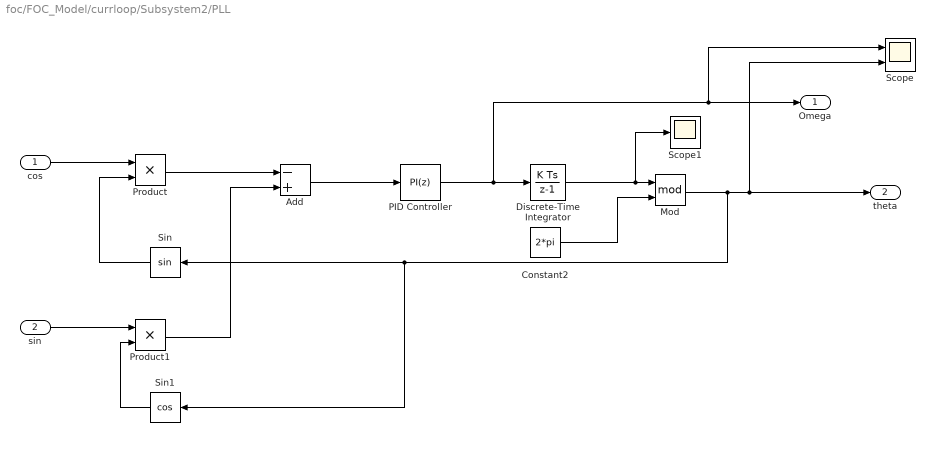
== system foc/FOC_Model/currloop/Subsystem2/PLL ==
  cos : Inport  OutDataTypeStr=single
  sin : Inport  Port=2  OutDataTypeStr=single
  Add : Sum  Inputs=-+
  Constant2 : Constant  Value=2*pi  OutDataTypeStr=single  SampleTime=Ts
  Discrete-Time Integrator : DiscreteIntegrator  SampleTime=Ts  ICPrevOutput=DiscIntNeverNeededParam  ICPrevScaledInput=DiscIntNeverNeededParam
  Mod : Math  Operator=mod  SignedPower=on  SaturateOnIntegerOverflow=on
  PID Controller : slpidlib/PID Controller  Controller=PI  Form=Parallel  TimeDomain=Discrete-time  UseExternalTs=off  SampleTime=-1  IntegratorMethod=Forward Euler  FilterMethod=Forward Euler  ControllerParametersSource=internal  P=22  I=400  D=0  UseFilter=on  N=100  TunerSelectOption=Transfer Function Based (PID Tuner App)  InitialConditionSource=internal  InitialConditionForIntegrator=0  InitialConditionForFilter=0  DifferentiatorICPrevScaledInput=0  ExternalReset=none  TrackingMode=off  Kt=1  LimitOutput=on  SatLimitsSource=internal  UpperSaturationLimit=3000  LowerSaturationLimit=-3000  LinearizeAsGain=on  AntiWindupMode=none  Kb=1  POutMin=[]  POutMax=[]  IOutMin=[]  IOutMax=[]  DOutMin=[]  DOutMax=[]  NOutMin=[]  NOutMax=[]  SumOutMin=[]  SumOutMax=[]  SaturationOutMin=[]  SaturationOutMax=[]  PParamMin=[]  PParamMax=[]  IParamMin=[]  IParamMax=[]  DParamMin=[]  DParamMax=[]  NParamMin=[]  NParamMax=[]  KbParamMin=[]  KbParamMax=[]  KtParamMin=[]  KtParamMax=[]  KbOutMin=[]  KbOutMax=[]  KtOutMin=[]  KtOutMax=[]  IntegratorOutMin=[]  IntegratorOutMax=[]  FilterOutMin=[]  FilterOutMax=[]  SumI1OutMin=[]  SumI1OutMax=[]  SumI2OutMin=[]  SumI2OutMax=[]  SumI3OutMin=[]  SumI3OutMax=[]  SumI4OutMin=[]  SumI4OutMax=[]  SumDOutMin=[]  SumDOutMax=[]  DifferentiatorOutMin=[]  DifferentiatorOutMax=[]  FilterDiffOutCoefMin=[]  FilterDiffOutCoefMax=[]  ReciprocalOutMin=[]  ReciprocalOutMax=[]  SumDenOutMin=[]  SumDenOutMax=[]  SumNumOutMin=[]  SumNumOutMax=[]  DivideOutMin=[]  DivideOutMax=[]  UdiffTsProdOutMin=[]  UdiffTsProdOutMax=[]  NTsProdOutMin=[]  NTsProdOutMax=[]  UintegralTsProdOutMin=[]  UintegralTsProdOutMax=[]  UngainTsProdOutMin=[]  UngainTsProdOutMax=[]  IntegratorContinuousStateAttributes=''  IntegratorStateMustResolveToSignalObject=off  IntegratorRTWStateStorageClass=Auto  FilterContinuousStateAttributes=''  FilterStateMustResolveToSignalObject=off  FilterRTWStateStorageClass=Auto  ParallelPVariant=InternalParameters  IdealPVariant=Disabled  IVariant=InternalParameters  DVariant=Disabled  IntegratorVariant=Discrete  SatVariant=Enabled  AWVariant=Passthrough  PCopyVariant=Disabled  TRVariant=Disabled  FdbkBlocksVariant=Forward  IdealPFdbkVariant=Disabled  SatFdbkVariant=Disabled  DerivativeFilterVariant=Disabled  NVariant=Disabled  NCopyVariant=Disabled_SignalSpec  FilterICVariant=Disabled  IntegratorICVariant=InternalICs  ExternalResetVariant=Disabled  TRSumVariant=Passthrough  SumFdbkVariant=Disabled  SumVariant=Sum_PI  TsampFilterVariant=InternalTs  TsampNgainVariant=Passthrough  TsampIntegralVariant=Passthrough  ExternalSaturationOutDataTypeStr=Inherit: Same as second input
  Product : Product
  Product1 : Product
  Scope : Scope  NumInputPorts=2
  Scope1 : Scope
  Sin : Trigonometry
  Sin1 : Trigonometry  Operator=cos
  Omega : Outport  OutDataTypeStr=single
  theta : Outport  Port=2  OutDataTypeStr=single
  wires:
  cos/1 -> Product/1
  Sin/1 -> Product/2
  Product/1 -> Add/1
  Add/1 -> PID Controller/1
  Product1/1 -> Add/2
  Sin1/1 -> Product1/2
  sin/1 -> Product1/1
  Constant2/1 -> Mod/2
  PID Controller/1 -> Scope/1, Omega/1, Discrete-Time Integrator/1
  Mod/1 -> Sin1/1, Sin/1, theta/1, Scope/2
  Discrete-Time Integrator/1 -> Scope1/1, Mod/1

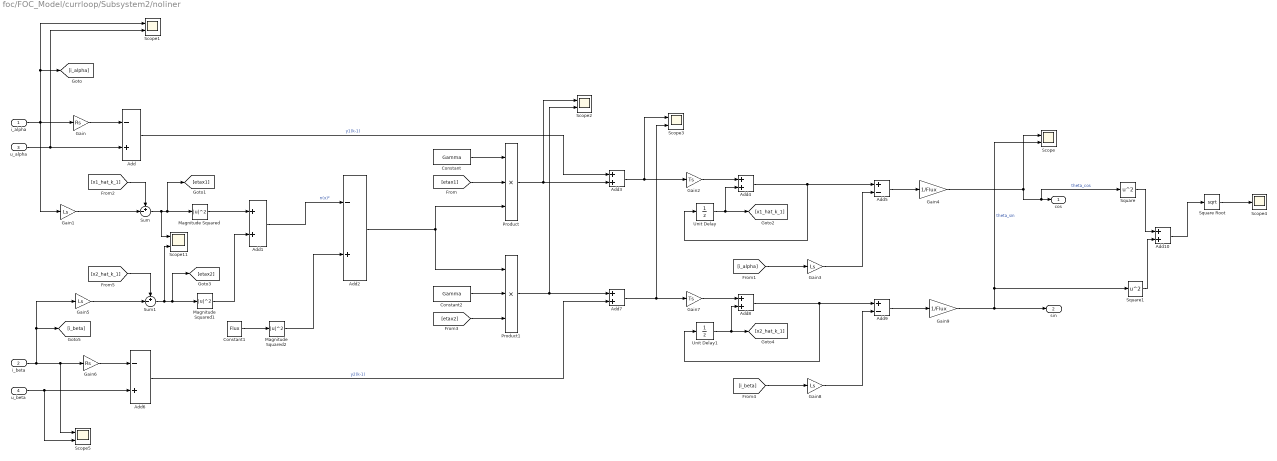
== system foc/FOC_Model/currloop/Subsystem2/noliner ==
  i_alpha : Inport  OutDataTypeStr=single
  i_beta : Inport  Port=2  OutDataTypeStr=single
  u_alpha : Inport  Port=3  OutDataTypeStr=single
  u_beta : Inport  Port=4  OutDataTypeStr=single
  Add : Sum  Inputs=-+
  Add1 : Sum  OutDataTypeStr=single
  Add{3..4,7..8,10} (5 alike) : Sum
  Add2 : Sum  Inputs=-+  OutDataTypeStr=single
  Add5 : Sum  Inputs=+-
  Add6 : Sum  Inputs=-+
  Add9 : Sum  Inputs=+-
  Constant : Constant  Value=Gamma
  Constant1 : Constant  Value=Flux  OutDataTypeStr=single
  Constant2 : Constant  Value=Gamma
  Gain : Gain  Gain=Rs
  Gain{1,3,5,8} (4 alike) : Gain  Gain=Ls
  Gain2 : Gain  Gain=Ts
  Gain4 : Gain  Gain=1/Flux
  Gain6 : Gain  Gain=Rs
  Gain7 : Gain  Gain=Ts
  Gain9 : Gain  Gain=1/Flux
  Magnitude Squared : Math  Operator=magnitude^2  SaturateOnIntegerOverflow=on
  Magnitude Squared1 : Math  Operator=magnitude^2  SaturateOnIntegerOverflow=on
  Magnitude Squared2 : Math  Operator=magnitude^2  SaturateOnIntegerOverflow=on
  Product : Product  Inputs=3
  Product1 : Product  Inputs=3
  Scope{,1..3,5,11} (6 alike) : Scope  NumInputPorts=2
  Scope4 : Scope
  Square : Math  Operator=square  SaturateOnIntegerOverflow=on
  Square Root : Sqrt  SaturateOnIntegerOverflow=on
  Square1 : Math  Operator=square  SaturateOnIntegerOverflow=on
  Sum : Sum  Inputs=+-|
  Sum1 : Sum  Inputs=+-|
  Unit Delay : UnitDelay  SampleTime=-1  HasFrameUpgradeWarning=on
  Unit Delay1 : UnitDelay  SampleTime=-1  HasFrameUpgradeWarning=on
  cos : Outport  OutDataTypeStr=single
  sin : Outport  Port=2  OutDataTypeStr=single
  wires:
  i_alpha/1 -> Gain/1, Scope1/1, [i_alpha], Gain1/1
  Gain/1 -> Add/1
  u_alpha/1 -> Scope1/2, Add/2
  Gain1/1 -> Sum/2
  Sum/1 -> Scope11/1, Magnitude Squared/1, [etax1]
  Magnitude Squared/1 -> Add1/1
  Add1/1 -> Add2/1  "n(x)²"
  Constant/1 -> Product/1
  [etax1] -> Product/2
  Add2/1 -> Product/3, Product1/1
  Product/1 -> Scope2/1, Add3/2
  Add/1 -> Add3/1  "y1(k-1)"
  Add3/1 -> Scope3/1, Gain2/1
  Gain2/1 -> Add4/1
  Unit Delay/1 -> [x1_hat_k_1], Add4/2
  Add4/1 -> Unit Delay/1, Add5/1
  [i_alpha] -> Gain3/1
  Gain3/1 -> Add5/2
  Add5/1 -> Gain4/1
  Gain5/1 -> Sum1/2
  Sum1/1 -> Scope11/2, Magnitude Squared1/1, [etax2]
  i_beta/1 -> Gain5/1, [i_beta], Scope5/1, Gain6/1
  Magnitude Squared1/1 -> Add1/2
  u_beta/1 -> Scope5/2, Add6/2
  Add6/1 -> Add7/2  "y2(k-1)"
  Gain6/1 -> Add6/1
  [x1_hat_k_1] -> Sum/1
  Constant1/1 -> Magnitude Squared2/1
  Magnitude Squared2/1 -> Add2/2
  Product1/1 -> Scope2/2, Add7/1
  Constant2/1 -> Product1/2
  [etax2] -> Product1/3
  Gain8/1 -> Add9/2
  [i_beta] -> Gain8/1
  Gain7/1 -> Add8/1
  Add8/1 -> Unit Delay1/1, Add9/1
  Add9/1 -> Gain9/1
  [x2_hat_k_1] -> Sum1/1
  Add7/1 -> Scope3/2, Gain7/1
  Unit Delay1/1 -> Add8/2, [x2_hat_k_1]
  Gain9/1 -> Square1/1, Scope/2, sin/1  "theta_sin"
  Gain4/1 -> Square/1, cos/1, Scope/1  "theta_cos"
  Square/1 -> Add10/1
  Square1/1 -> Add10/2
  Add10/1 -> Square Root/1
  Square Root/1 -> Scope4/1

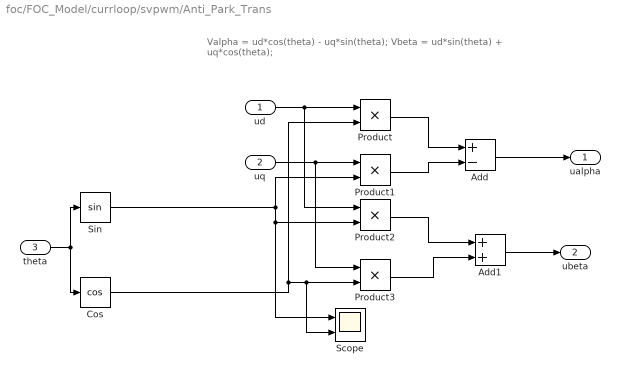
== system foc/FOC_Model/currloop/svpwm/Anti_Park_Trans ==
  note: Valpha = ud*cos(theta) - uq*sin(theta);
      | Vbeta = ud*sin(theta) + uq*cos(theta);
  ud : Inport  OutDataTypeStr=single
  uq : Inport  Port=2  OutDataTypeStr=single
  theta : Inport  Port=3
  Add : Sum  Inputs=+-
  Add1 : Sum
  Cos : Trigonometry  Operator=cos
  Product{,1..3} (4 alike) : Product
  Scope : Scope  NumInputPorts=2
  Sin : Trigonometry
  ualpha : Outport  OutDataTypeStr=single
  ubeta : Outport  Port=2  OutDataTypeStr=single
  wires:
  Add/1 -> ualpha/1
  ud/1 -> Product2/1, Product/1
  Cos/1 -> Product/2, Scope/2, Product3/2
  Product/1 -> Add/1
  uq/1 -> Product3/1, Product1/1
  theta/1 -> Sin/1, Cos/1
  Product1/1 -> Add/2
  Product2/1 -> Add1/1
  Product3/1 -> Add1/2
  Add1/1 -> ubeta/1
  Sin/1 -> Scope/1, Product2/2, Product1/2

== matlab function foc/FOC_Model/currloop/svpwm/foc ==
  data: Valpha input; Tcmp1 output; Vbeta input; Udc input; Tpwm input; Tcmp2 output; Tcmp3 output; sector output
function [Tcmp1,Tcmp2,Tcmp3,sector] = fcn(Valpha,Vbeta,Udc,Tpwm)
%#codegen

sector = single(0);
Tcmp1 = single(0);
Tcmp2 = single(0);
Tcmp3 = single(0);

%========Parameters statement================

    Vref1 = Vbeta;							                   
    Vref2 = (sqrt(3)*Valpha - Vbeta)/2; 				    
    Vref3 = (-sqrt(3)*Valpha - Vbeta)/2;					
   
 %========Sector calculation=================

  if (Vref1>0)
	   sector = single(1);
  end
  if (Vref2>0)
	   sector = sector+single(2);
  end
  if (Vref3>0)
       sector = sector+single(4);
  end

%======== X Y Z calculation===================

X = sqrt(3)*Vbeta*Tpwm/Udc;
Y = Tpwm/Udc*(3/2*Valpha+sqrt(3)/2*Vbeta);
Z = Tpwm/Udc*(-3/2*Valpha+sqrt(3)/2*Vbeta);	         

%==========Duty ratio calculation================
switch (sector)   
    case 1
        T1 = Z; T2 = Y; 
	case 2
        T1 = Y; T2 = -X; 
	case 3
        T1 = -Z; T2 = X; 
	case 4
        T1 = -X; T2 = Z;
	case 5
        T1 = X; T2 = -Y;
    otherwise
        T1 = -Y; T2 = -Z;
end

if T1+T2 > Tpwm
    T1 = T1/(T1+T2);
    T2 = T2/(T1+T2);
else
    T1 = T1;
    T2 = T2;
end
ta = (Tpwm-(T1+T2))/4.0;
tb = ta+T1/2;
tc = tb+T2/2;

%==========Duty ratio calculation================
switch (sector)
    case 1 
        Tcmp1=tb;
        Tcmp2=ta;
        Tcmp3=tc; 
        
    case 2 
        Tcmp1=ta;
        Tcmp2=tc;
        Tcmp3=tb; 
       
    case 3 
        Tcmp1=ta;
        Tcmp2=tb;
        Tcmp3=tc; 
        
    case 4 
        Tcmp1=tc;
        Tcmp2=tb;
        Tcmp3=ta;
        
    case 5 
        Tcmp1=tc;
        Tcmp2=ta;
        Tcmp3=tb;
        
   case 6
       Tcmp1=tb;
       Tcmp2=tc;
       Tcmp3=ta;
end
end

== stateflow chart foc/FOC_Model/motor_state/Chart1 ==
  state IDLE
    Motor_state = 1;
    soure=0;
  state AlignStage
    Motor_state = 2;
    soure=0;
  state RunStage
    Motor_state = 3;
    soure=1;
  (default) -> IDLE
  IDLE -> AlignStage : [Motor_OnOff ==1]
  AlignStage -> RunStage [order 1] : [after(0.1,sec)]
  RunStage -> IDLE : [Motor_OnOff ==0]
  AlignStage -> IDLE [order 2] : [Motor_OnOff == 0]
  data: Motor_OnOff input; Motor_state output; soure output single
